simulink model "D_LowerandMore_OutputWaterFlow"  (R2016a)
settings: Solver=VariableStepAuto  StartTime=0.0  StopTime=10.0  MaxStep=1e-3  RelTol=1e-3
InitFcn:
  | S1=20;
  | S2=20;
  | h1=5;
  | h2=5;
settings Model: Creator=Hossein  LastModifiedBy=Hossein

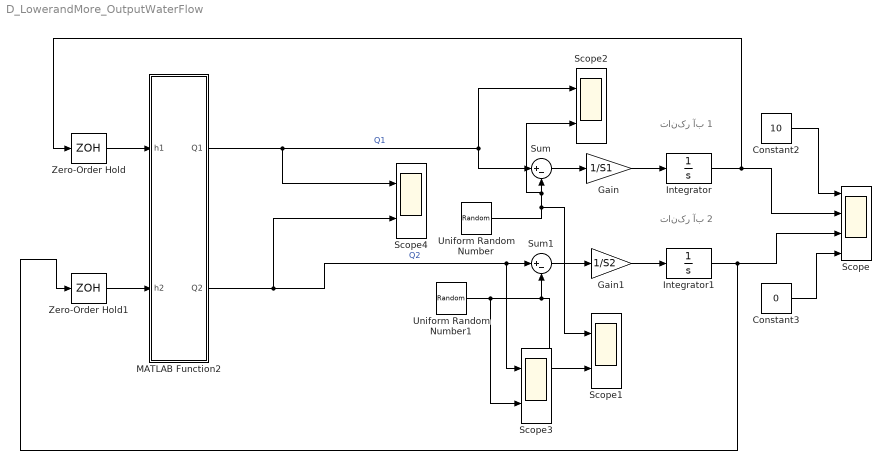
== system D_LowerandMore_OutputWaterFlow ==
  note: تانکر آب 1
  note: تانکر آب 2
  Constant2 : Constant  Value=10
  Constant3 : Constant  Value=0
  Gain : Gain  Gain=1/S1
  Gain1 : Gain  Gain=1/S2
  Integrator : Integrator  InitialCondition=h1
  Integrator1 : Integrator  InitialCondition=h2
  MATLAB Function2 : MATLAB Function  TreatAsAtomicUnit=on
  Scope : Scope  NumInputPorts=4
  Scope{1..4} (4 alike) : Scope  NumInputPorts=2
  Sum : Sum  Inputs=|+-
  Sum1 : Sum  Inputs=|+-
  Uniform Random Number : UniformRandomNumber  Minimum=30  Maximum=36  Seed=randi([1,5])  SampleTime=2
  Uniform Random Number1 : UniformRandomNumber  Minimum=23  Maximum=32  Seed=randi([1,5])  SampleTime=0.3
  Zero-Order Hold : ZeroOrderHold  SampleTime=0.01
  Zero-Order Hold1 : ZeroOrderHold  SampleTime=0.01
  wires:
  MATLAB Function2/1(Q1) -> Scope4/1, Sum/1, Scope2/1  "Q1"
  MATLAB Function2/2(Q2) -> Scope4/2, Scope3/1, Sum1/1  "Q2"
  Sum/1 -> Gain/1
  Gain/1 -> Integrator/1
  Gain1/1 -> Integrator1/1
  Sum1/1 -> Gain1/1
  Integrator/1 -> Zero-Order Hold/1, Scope/2
  Integrator1/1 -> Zero-Order Hold1/1, Scope/3
  Constant2/1 -> Scope/1
  Constant3/1 -> Scope/4
  Uniform Random Number/1 -> Scope1/1, Scope2/2, Sum/2
  Uniform Random Number1/1 -> Scope3/2, Scope1/2, Sum1/2
  Zero-Order Hold/1 -> MATLAB Function2/1(h1)
  Zero-Order Hold1/1 -> MATLAB Function2/2(h2)

== matlab function D_LowerandMore_OutputWaterFlow/MATLAB Function2 ==
  data: h1 input; Q1 output; Q2 output; h2 input
function [Q1,Q2] = fcn(h1,h2)
%#codegen
    % Q is Q1
     persistent q1 


     if isempty(q1)
         q1=30; 
     end
    
 Q1=q1;
    if h1>h2
        Q1=Q1*0.996;
    else
        Q1=Q1*1.004;
    end
 q1=Q1;
 Q2=70-q1;
